simulink model "PIDOVI"  (R2021a)
settings: Solver=FixedStepAuto  StartTime=0.0  StopTime=1000.0  FixedStep=0.1  RelTol=1e-3
libraries: fuzblock x2
settings Model: Creator=Ivan  LastModifiedBy=Ivan

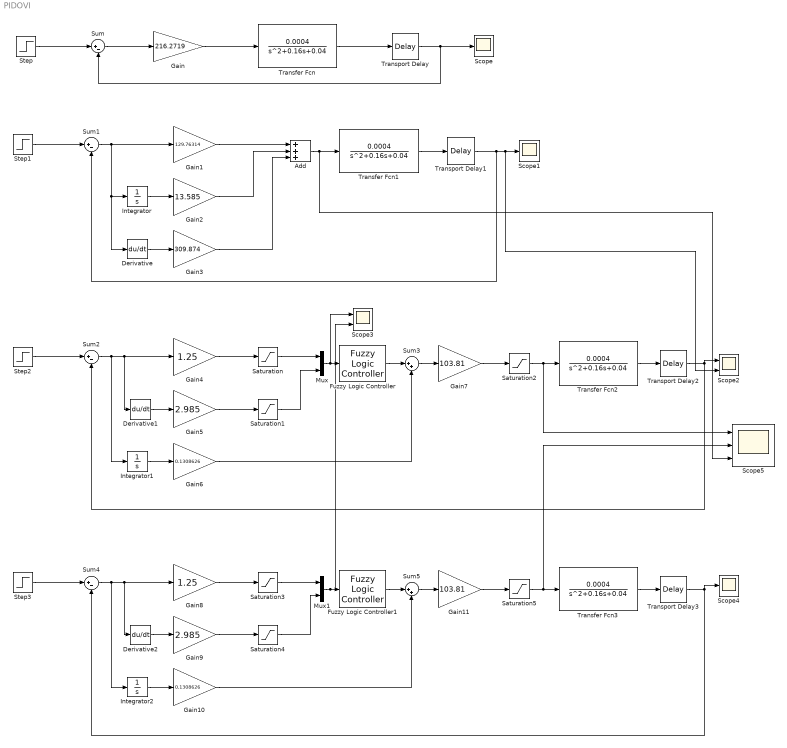
== system PIDOVI ==
  Add : Sum  Inputs=+++
  Derivative : Derivative
  Derivative1 : Derivative
  Derivative2 : Derivative
  Fuzzy Logic Controller : fuzblock/Fuzzy Logic  Controller  FIS='MASINA.fis'  OutputSampleNumber=101  DataType=double  FuzzifiedInputs=off  RuleFiringStrengths=off  RuleOutputs=off  AggregatedOutputs=off  SimulateUsing=Interpreted execution  OutOfRangeInputValueMessage=warning  NoRuleFiredMessage=warning  EmptyOutputFuzzySetMessage=warning
  Fuzzy Logic Controller1 : fuzblock/Fuzzy Logic  Controller  FIS='NELINEARNO.fis'  OutputSampleNumber=101  DataType=double  FuzzifiedInputs=off  RuleFiringStrengths=off  RuleOutputs=off  AggregatedOutputs=off  SimulateUsing=Interpreted execution  OutOfRangeInputValueMessage=warning  NoRuleFiredMessage=warning  EmptyOutputFuzzySetMessage=warning
  Gain : Gain  Gain=216.2719
  Gain1 : Gain  Gain=129.76314
  Gain10 : Gain  Gain=0.1308626
  Gain11 : Gain  Gain=103.81
  Gain2 : Gain  Gain=13.585
  Gain3 : Gain  Gain=309.874
  Gain4 : Gain  Gain=1.25
  Gain5 : Gain  Gain=2.985
  Gain6 : Gain  Gain=0.1308626
  Gain7 : Gain  Gain=103.81
  Gain8 : Gain  Gain=1.25
  Gain9 : Gain  Gain=2.985
  Integrator : Integrator
  Integrator1 : Integrator
  Integrator2 : Integrator
  Mux : Mux  Inputs=2
  Mux1 : Mux  Inputs=2
  Saturation{,1,3..4} (4 alike) : Saturate  UpperLimit=1  LowerLimit=-1
  Saturation2 : Saturate  UpperLimit=100  LowerLimit=-100
  Saturation5 : Saturate  UpperLimit=100  LowerLimit=-100
  Scope : Scope
  Scope1 : Scope
  Scope2 : Scope  NumInputPorts=2
  Scope3 : Scope  NumInputPorts=2
  Scope4 : Scope
  Scope5 : Scope  NumInputPorts=3
  Step{,1..3} (4 alike) : Step  Time=500  SampleTime=0
  Sum{,1..2,4} (4 alike) : Sum  Inputs=|+-
  Sum3 : Sum  Inputs=|++
  Sum5 : Sum  Inputs=|++
  Transfer Fcn{,1..3} (4 alike) : TransferFcn  Numerator=[0.0004]  Denominator=[1 0.16 0.04]
  Transport Delay{,1..3} (4 alike) : TransportDelay  DelayTime=2
  wires:
  Step/1 -> Sum/1
  Sum/1 -> Gain/1
  Gain/1 -> Transfer Fcn/1
  Transfer Fcn/1 -> Transport Delay/1
  Transport Delay/1 -> Sum/2, Scope/1
  Step1/1 -> Sum1/1
  Sum1/1 -> Derivative/1, Integrator/1, Gain1/1
  Integrator/1 -> Gain2/1
  Derivative/1 -> Gain3/1
  Gain1/1 -> Add/1
  Gain2/1 -> Add/2
  Gain3/1 -> Add/3
  Add/1 -> Scope5/3, Transfer Fcn1/1
  Transfer Fcn1/1 -> Transport Delay1/1
  Transport Delay1/1 -> Scope2/2, Scope1/1, Sum1/2
  Transport Delay2/1 -> Sum2/2, Scope2/1
  Integrator1/1 -> Gain6/1
  Gain6/1 -> Sum3/2
  Gain4/1 -> Saturation/1
  Gain5/1 -> Saturation1/1
  Step2/1 -> Sum2/1
  Mux/1 -> Scope3/1, Fuzzy Logic Controller/1
  Saturation/1 -> Mux/1
  Saturation1/1 -> Mux/2
  Fuzzy Logic Controller/1 -> Sum3/1
  Sum3/1 -> Gain7/1
  Gain7/1 -> Saturation2/1
  Saturation2/1 -> Scope5/1, Transfer Fcn2/1
  Transfer Fcn2/1 -> Transport Delay2/1
  Derivative1/1 -> Gain5/1
  Sum2/1 -> Integrator1/1, Derivative1/1, Gain4/1
  Sum5/1 -> Gain11/1
  Sum4/1 -> Integrator2/1, Derivative2/1, Gain8/1
  Transfer Fcn3/1 -> Transport Delay3/1
  Saturation4/1 -> Mux1/2
  Saturation3/1 -> Mux1/1
  Transport Delay3/1 -> Scope4/1, Sum4/2
  Gain9/1 -> Saturation4/1
  Fuzzy Logic Controller1/1 -> Sum5/1
  Mux1/1 -> Scope3/2, Fuzzy Logic Controller1/1
  Gain11/1 -> Saturation5/1
  Step3/1 -> Sum4/1
  Gain10/1 -> Sum5/2
  Gain8/1 -> Saturation3/1
  Derivative2/1 -> Gain9/1
  Integrator2/1 -> Gain10/1
  Saturation5/1 -> Scope5/2, Transfer Fcn3/1
